simulink model "BuckBoostMPPT"  (R2023a)
settings: Solver=VariableStepAuto  StartTime=0.0  StopTime=10.0  RelTol=1e-3
libraries: spsSeriesRLCBranchLib x4, SignalEditorBlockLib x2, spsVoltageMeasurementLib x2, spsCurrentMeasurementLib x1, spsDiodeLib x1, spsIGBTLib x1, spsPVArrayLib x1, spsPWMGeneratorDCDCLib x1, spspowerguiLib x1
settings Model: Creator=prakrgh  LastModifiedBy=prakrgh

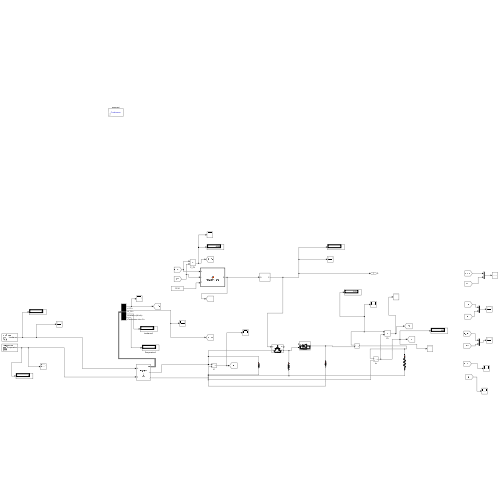
[thumbnail: Simulink's stored preview of the top-level diagram]
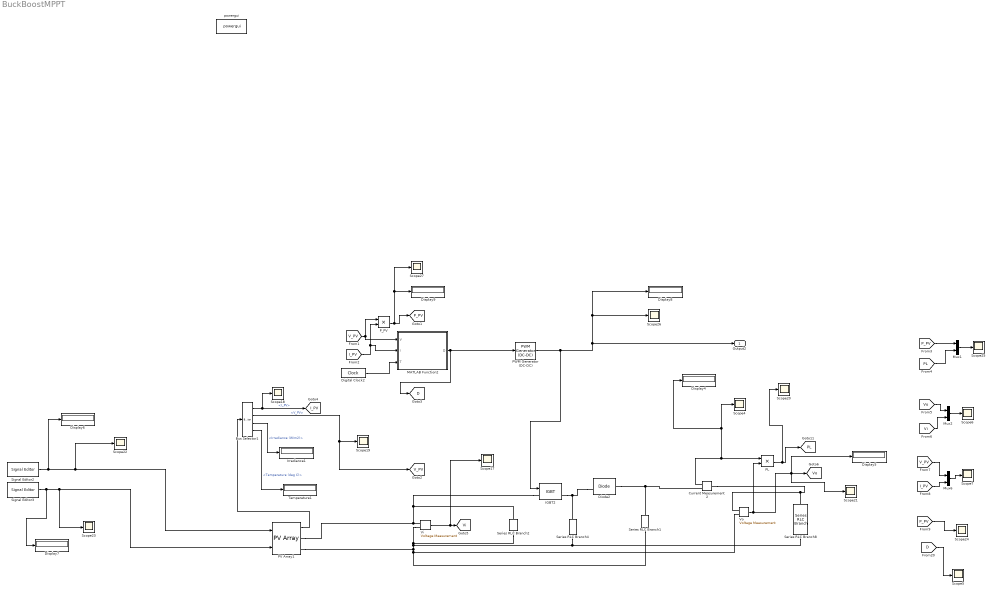
== system BuckBoostMPPT ==
  Bus Selector1 : BusSelector  OutputSignals=I_PV,V_PV,Irradiance (W/m2),Temperature (deg C)
  Current Measurement2 : spsCurrentMeasurementLib/Current Measurement  PhasorSimulation=off  OutputType=Complex  PSBequivalent=0
  Digital Clock2 : DigitalClock
  Diode2 : spsDiodeLib/Diode  Ron=0.001  Lon=0  Vf=0.8  IC=0  UseSnubber=0  Rs=500  Cs=250e-9  Measurements=on
  Display{4..9} (6 alike) : Display
  IGBT2 : spsIGBTLib/IGBT  Ron=0.001  Lon=0  Vf=1  Tf=1e-6  Tt=2e-6  IC=0  Rs=1e5  Cs=inf  Measurements=on
  Irradiance1 : Display
  MATLAB Function2 : MATLAB Function  TreatAsAtomicUnit=on
  Mux1 : Mux  Inputs=2
  Mux2 : Mux  Inputs=2
  Mux6 : Mux  Inputs=2
  PL : Product
  PV Array1 : spsPVArrayLib/PV Array  Npar=40  Nser=10  PlotType=array @ 1000 W/m2 & specified temperatures  S_vec="[ 1000  500  100 ]"  Temp_C_vec="[ 45 25  ]"  ModuleName=User-defined  PlotWhenSelected=off  Pm=465.0328  Ncell=72  Voc=50.15  Isc=11.49  Vm=42.43  Im=10.96  beta_Voc_pc=-0.272  alpha_Isc_pc=0.044  beta_Voc=-0.13641  alpha_Isc=0.0050556  IL=11.5368  I0=1.1543e-11  nI=0.98156  Rsh=405.7878  Rs=0.18205  RobustModel=off  RobustCellTemperature=313.3991  BAL=off  Tc=1e-6  Tfilter=5e-5
  PWM Generator (DC-DC) : spsPWMGeneratorDCDCLib/PWM Generator (DC-DC)  Fsw=5000  Ts=0
  P_PV : Product
  Scope{4..7,17..27} (15 alike) : Scope
  Series RLC Branch1 : spsSeriesRLCBranchLib/Series RLC Branch  LConnTagsString=__new0  RConnTagsString=__new0  BranchType=C  Resistance=1  Inductance=1e-3  SetiL0=off  InitialCurrent=0  Capacitance=1.41e-3  Setx0=off  InitialVoltage=0  Measurements=None
  Series RLC Branch2 : spsSeriesRLCBranchLib/Series RLC Branch  LConnTagsString=__new0  RConnTagsString=__new0  BranchType=C  Resistance=1  Inductance=1e-3  SetiL0=off  InitialCurrent=0  Capacitance=0.305  Setx0=off  InitialVoltage=0  Measurements=None
  Series RLC Branch4 : spsSeriesRLCBranchLib/Series RLC Branch  LConnTagsString=__new0  RConnTagsString=__new0  BranchType=L  Resistance=1  Inductance=0.920e-3  SetiL0=off  InitialCurrent=0  Capacitance=1e-6  Setx0=off  InitialVoltage=0  Measurements=None
  Series RLC Branch8 : spsSeriesRLCBranchLib/Series RLC Branch  LConnTagsString=__new0  RConnTagsString=__new0  BranchType=R  Resistance=79.180  Inductance=1e-3  SetiL0=off  InitialCurrent=0  Capacitance=1e-6  Setx0=off  InitialVoltage=0  Measurements=None
  Signal Editor2 : SignalEditorBlockLib/Signal Editor  FileName=IrradianceTemperature.mat  ActiveScenario=Irradiance  ActiveSignal=Irradiance  IsBus=off  OutputBusObjectStr=Bus: BusObject  SampleTime=0  Interpolate=off  ZeroCross=off  OutputAfterFinalValue=Setting to zero  Unit=W  PreserveSignalName=on  ApplySigPropsToAllScenarios=on
  Signal Editor3 : SignalEditorBlockLib/Signal Editor  FileName=IrradianceTemperature.mat  ActiveScenario=Temperature  ActiveSignal=Temperature  IsBus=off  OutputBusObjectStr=Bus: BusObject  SampleTime=0  Interpolate=off  ZeroCross=off  OutputAfterFinalValue=Setting to zero  Unit=K  PreserveSignalName=on  ApplySigPropsToAllScenarios=on
  Temperature1 : Display
  Vi : spsVoltageMeasurementLib/Voltage Measurement  PhasorSimulation=off  OutputType=Complex  PSBequivalent=0
  Vo : spsVoltageMeasurementLib/Voltage Measurement  PhasorSimulation=off  OutputType=Complex  PSBequivalent=0
  powergui : spspowerguiLib/powergui  Priority=1  SimulationMode=Continuous  SampleTime=1e-06  frequency=60  Iterations=50  frequencyindice=0  Pbase=100e6  ErrMax=1e-4  UnitsV=kV  UnitsW=MW  buscounter=0  FunctionMessages=off  echomessages=off  EnableUseOfTLC=off  CurrentSourceSwitches=off  DisableSnubberDevices=off  DisableRonSwitches=off  DisableVfSwitches=off  DisplayEquations=off  AutomaticDiscreteSolvers=on  SolverType=Tustin/Backward Euler (TBE)  Interpol=off  ExternalGateDelay=off  methode=off  Ts=100  x0status=blocks  SPID=on  SwTol=0  HookPort=off  NonlinearTolerance=1e-4  nMaxIteration=100  ContinueOnMaxIteration=off  RestoreLinks=warning  ResistiveCurrentMeasurement=off  Frange=[0:2:500]  Ylog=off  Xlog=on  ShowGrid=off  save=off  variable=ZData  structure=0  ZoomFFT=off  StartTime=0.0  cycles=1  DisplayStyle=1  fundamental=60  FreqAxis=off  MaxFrequency=1000  frequencyindicesteady=1  RmsSteady=1  display=off
  Output2 : Outport  SignalName=G
  tag scope: D=global, I_PV=global, PL=global, P_PV=global, V_PV=global, Vi=global, Vo=global
  wires:
  [P_PV] -> Scope24/1
  PWM Generator (DC-DC)/1 -> IGBT2/1, Output2/1, Scope26/1, Display8/1
  [I_PV] -> Mux6/2
  Digital Clock2/1 -> MATLAB Function2/3(T)
  Bus Selector1/3 -> Irradiance1/1  "<Irradiance (W/m2)>"
  Current Measurement2/1 -> Display4/1, Scope4/1, PL/1
  Bus Selector1/4 -> Temperature1/1  "<Temperature (deg C)>"
  Mux2/1 -> Scope6/1
  Bus Selector1/1 -> [I_PV], Scope18/1  "<I_PV>"
  PV Array1/1 -> Bus Selector1/1
  [P_PV] -> Mux1/1
  [V_PV] -> Mux6/1
  [I_PV] -> P_PV/2, MATLAB Function2/2(I)
  Mux6/1 -> Scope7/1
  MATLAB Function2/1(D) -> [D], PWM Generator (DC-DC)/1
  [Vi] -> Mux2/2
  P_PV/1 -> Display9/1, Scope27/1, [P_PV]
  Signal Editor2/1 -> PV Array1/1, Scope22/1, Display6/1
  [V_PV] -> MATLAB Function2/1(V), P_PV/1
  [Vo] -> Mux2/1
  [D] -> Scope5/1
  PL/1 -> Scope20/1, [PL]
  Vo/1 -> Display5/1, Scope21/1, [Vo], PL/2
  Vi/1 -> Scope17/1, [Vi]
  Bus Selector1/2 -> [V_PV], Scope19/1  "<V_PV>"
  [PL] -> Mux1/2
  Signal Editor3/1 -> PV Array1/2, Scope23/1, Display7/1
  Mux1/1 -> Scope25/1
  connections:
  Vi/LConn2 -- Series RLC Branch1/RConn1 -- Vo/LConn1 -- PV Array1/RConn2 -- Series RLC Branch8/RConn1 -- Series RLC Branch4/RConn1 -- Series RLC Branch2/RConn1
  Vo/LConn2 -- Current Measurement2/LConn1 -- Series RLC Branch8/LConn1
  Current Measurement2/RConn1 -- Diode2/LConn1 -- Series RLC Branch1/LConn1
  Diode2/RConn1 -- IGBT2/RConn1 -- Series RLC Branch4/LConn1
  IGBT2/LConn1 -- Vi/LConn1 -- PV Array1/RConn1 -- Series RLC Branch2/LConn1

== matlab function BuckBoostMPPT/MATLAB Function2 ==
  settings: updateMethod=DISCRETE
  data: V input; D output; I input; T input
function D = PerturbObserve(V , I , T)

persistent  Pold P dP d deltaD n m ;

if isempty(n)
    n=1 ; d=1 ; Pold=0;V = 30 ;I=0; deltaD=0.01;dP=0;P=0;m=0;
end

if (T > n*0.02)
    n = n + 1;
    Pold = P ;
    P = V*I;
    dP = P - Pold ;
    if (m==0)
        if dP > 1
            m = 1;
            d = d + deltaD;
        else 
            if dP < -1 
                m = 1;
                d = d - deltaD;
            else 
                m = 0;
            end 
        end 
    else 
        if ((dP<1)&&(dP>-1))
            m=0;
            d=d;
        else 
            if ((dP/deltaD)>0)
                m=1;
                d=d+deltaD;
            else 
                m=1;
                d=d-deltaD;
            end
        end
    end
end 
D=d/(d+1);
if D <0.1
    D=0.1;
    d= D/(1-D);
else 
    if D> 0.9 
        D = 0.9;
        d = D / (1-D);
    else 
    end 
end
